simulink model "SLDVBlocks1"  (R2017b)
settings: Solver=FixedStepDiscrete  StartTime=0.0  StopTime=19.8  FixedStep=0.200000  RelTol=1e-3
libraries: simulink x10
settings Model: Creator=hbourbou  LastModifiedBy=hbourbou
settings DataIOCC: ExternalInput=input_dataset  LoadExternalInput=on  SaveState=on
settings DebuggingCC: AlgebraicLoopMsg=error
settings GRTTargetCC: ExtMode=on

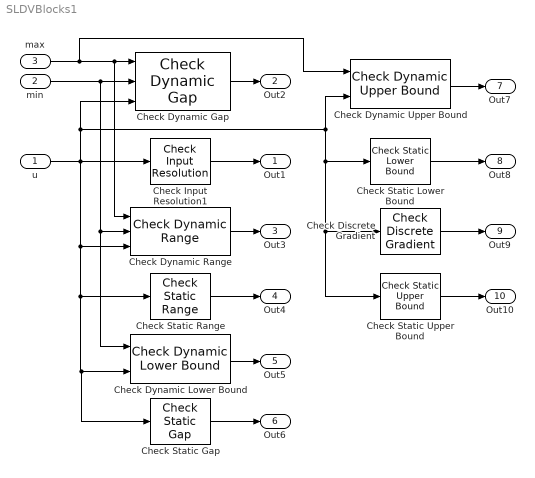
== system SLDVBlocks1 ==
  u : Inport
  min : Inport  Port=2
  max : Inport  Port=3
  Check Discrete Gradient : simulink/Model Verification/Check Discrete Gradient  Description=| du / dt | < 1  gradient=1  enabled=on  stopWhenAssertionFail=off  export=on  icon=graphic
      settings: SourceProductName=Simulink  SourceProductBaseCode=SL
  Check Dynamic Gap : simulink/Model Verification/Check  Dynamic Gap  Description=u < min || max < u  enabled=on  stopWhenAssertionFail=off  export=on  icon=graphic
      settings: SourceProductName=Simulink  SourceProductBaseCode=SL
  Check Dynamic Range : simulink/Model Verification/Check  Dynamic Range  Description=min < u < max  enabled=on  callback=""  stopWhenAssertionFail=off  export=on  icon=graphic
      settings: SourceProductName=Simulink  SourceProductBaseCode=SL
  Check Static Gap : simulink/Model Verification/Check  Static Gap  Description=u <= 0 || 100 <= u  max=100  max_included=on  min=0  min_included=on  enabled=on  stopWhenAssertionFail=off  export=on  icon=graphic
      settings: SourceProductName=Simulink  SourceProductBaseCode=SL
  Check Static Range : simulink/Model Verification/Check  Static Range  Description=0 <= u <= 100  max=100  max_included=on  min=0  min_included=on  enabled=on  stopWhenAssertionFail=off  export=on  icon=graphic
      settings: SourceProductName=Simulink  SourceProductBaseCode=SL
  Check Dynamic Lower Bound : simulink/Model Verification/Check Dynamic  Lower Bound  Description=min < u  Enabled=on  stopWhenAssertionFail=off  export=on  icon=graphic
      settings: SourceProductName=Simulink  SourceProductBaseCode=SL
  Check Dynamic Upper Bound : simulink/Model Verification/Check Dynamic  Upper Bound  Description=u < max  enabled=on  stopWhenAssertionFail=off  export=on  icon=graphic
      settings: SourceProductName=Simulink  SourceProductBaseCode=SL
  Check Input Resolution1 : simulink/Model Verification/Check Input  Resolution  Description=-Inf < u < +Inf  resolution=1  enabled=on  stopWhenAssertionFail=off  export=on
      settings: SourceProductName=Simulink  SourceProductBaseCode=SL
  Check Static Lower Bound : simulink/Model Verification/Check Static  Lower Bound  Description=0 <= u  min=0  min_included=on  enabled=on  stopWhenAssertionFail=off  export=on  icon=graphic
      settings: SourceProductName=Simulink
  Check Static Upper Bound : simulink/Model Verification/Check Static  Upper Bound  Description=u <= 0  max=0  max_included=on  enabled=on  stopWhenAssertionFail=off  export=on  icon=graphic
      settings: SourceProductName=Simulink  SourceProductBaseCode=SL
  Out1 : Outport
  Out2 : Outport  Port=2
  Out3 : Outport  Port=3
  Out4 : Outport  Port=4
  Out5 : Outport  Port=5
  Out6 : Outport  Port=6
  Out7 : Outport  Port=7
  Out8 : Outport  Port=8
  Out9 : Outport  Port=9
  Out10 : Outport  Port=10
  wires:
  Check Input Resolution1/1 -> Out1/1
  u/1 -> Check Input Resolution1/1, Check Static Gap/1, Check Dynamic Lower Bound/2, Check Static Range/1, Check Dynamic Range/3, Check Dynamic Upper Bound/2, Check Static Upper Bound/1, Check Discrete Gradient/1, Check Static Lower Bound/1, Check Dynamic Gap/3
  max/1 -> Check Dynamic Upper Bound/1, Check Dynamic Range/1, Check Dynamic Gap/1
  min/1 -> Check Dynamic Lower Bound/1, Check Dynamic Range/2, Check Dynamic Gap/2
  Check Dynamic Gap/1 -> Out2/1
  Check Dynamic Range/1 -> Out3/1
  Check Static Range/1 -> Out4/1
  Check Dynamic Lower Bound/1 -> Out5/1
  Check Static Gap/1 -> Out6/1
  Check Dynamic Upper Bound/1 -> Out7/1
  Check Static Lower Bound/1 -> Out8/1
  Check Discrete Gradient/1 -> Out9/1
  Check Static Upper Bound/1 -> Out10/1
